simulink library "roller485lib"  (R2023a)
settings: Solver=VariableStepAuto  StartTime=0.0  StopTime=10.0  RelTol=1e-3
libraries: arduinolib x173, simulink x66
(part 5 of 6)

== system roller485lib/I2C Write/relative angle command [deg]/Enabled Subsystem (PID setting) ==
  P : Inport
  I : Inport  Port=2
  D : Inport  Port=3
  Enable : EnablePort
  " x 10^5 " : Gain  Gain=1e5
  Data Type Conversion1 : DataTypeConversion  OutDataTypeStr=uint32  SaturateOnIntegerOverflow=off  RndMeth=Floor
  Data Type Conversion2 : DataTypeConversion  OutDataTypeStr=uint32  SaturateOnIntegerOverflow=off  RndMeth=Floor
  Data Type Conversion3 : DataTypeConversion  OutDataTypeStr=uint32  SaturateOnIntegerOverflow=off  RndMeth=Floor
  I2C Write (0xA0) : arduinolib/I2C Write  I2CModule=0  Mode=Master  SlaveAddress=I2CAddress  SlaveByteOrder=LittleEndian  Direction=Transmitter  RegisterAddressMode=on  RegisterAddress=0xA0  SlaveDataType=uint8  DataLength=1  NoAck=off  RepeatedStart=off  OutputStatus=off  blockPlatform=ARDUINO
  I2C Write (0xA4) : arduinolib/I2C Write  I2CModule=0  Mode=Master  SlaveAddress=I2CAddress  SlaveByteOrder=LittleEndian  Direction=Transmitter  RegisterAddressMode=on  RegisterAddress=0xA4  SlaveDataType=uint8  DataLength=1  NoAck=off  RepeatedStart=off  OutputStatus=off  blockPlatform=ARDUINO
  I2C Write (0xA8) : arduinolib/I2C Write  I2CModule=0  Mode=Master  SlaveAddress=I2CAddress  SlaveByteOrder=LittleEndian  Direction=Transmitter  RegisterAddressMode=on  RegisterAddress=0xA8  SlaveDataType=uint8  DataLength=1  NoAck=off  RepeatedStart=off  OutputStatus=off  blockPlatform=ARDUINO
  x 10^5 : Gain  Gain=1e5
  x 10^7 : Gain  Gain=1e7
  wires:
  P/1 -> x 10^5/1
  I/1 -> x 10^7/1
  D/1 -> " x 10^5 "/1
  Data Type Conversion2/1 -> I2C Write (0xA4)/1
  Data Type Conversion3/1 -> I2C Write (0xA8)/1
  Data Type Conversion1/1 -> I2C Write (0xA0)/1
  x 10^5/1 -> Data Type Conversion1/1
  x 10^7/1 -> Data Type Conversion2/1
  " x 10^5 "/1 -> Data Type Conversion3/1

== system roller485lib/I2C Write/relative angle command [deg]/Enabled Subsystem (initialization angle) ==
  Enable : EnablePort
  Data Type Conversion : DataTypeConversion  OutDataTypeStr=double  SaturateOnIntegerOverflow=off  RndMeth=Floor
  I2C Read (0x90) : arduinolib/I2C Read  I2CModule=0  Mode=Master  SlaveAddress=I2CAddress  SlaveByteOrder=LittleEndian  Direction=Receiver  RegisterAddressMode=on  RegisterAddress=0x90  SlaveDataType=int32  DataLength=1  NoAck=off  RepeatedStart=off  OutputStatus=off  blockPlatform=ARDUINO  SampleTime=sample_time
  x (1/100) : Gain  Gain=1/100
  initial angle : Outport
  wires:
  I2C Read (0x90)/1 -> Data Type Conversion/1
  Data Type Conversion/1 -> x (1/100)/1
  x (1/100)/1 -> initial angle/1

== system roller485lib/I2C Write/relative angle command [deg]/Enabled Subsystem (mode setting) ==
  mode : Inport
  Enable : EnablePort
  Data Type Conversion : DataTypeConversion  OutDataTypeStr=uint8  SaturateOnIntegerOverflow=off  RndMeth=Floor
  I2C Write (0x01) : arduinolib/I2C Write  I2CModule=0  Mode=Master  SlaveAddress=I2CAddress  SlaveByteOrder=BigEndian  Direction=Transmitter  RegisterAddressMode=on  RegisterAddress=0x01  SlaveDataType=uint8  DataLength=1  NoAck=off  RepeatedStart=off  OutputStatus=off  blockPlatform=ARDUINO
  wires:
  Data Type Conversion/1 -> I2C Write (0x01)/1
  mode/1 -> Data Type Conversion/1

== system roller485lib/I2C Write/relative angle command [deg] and max current [mA]/Enabled Subsystem (PID setting) ==
  P : Inport
  I : Inport  Port=2
  D : Inport  Port=3
  Enable : EnablePort
  " x 10^5 " : Gain  Gain=1e5
  Data Type Conversion1 : DataTypeConversion  OutDataTypeStr=uint32  SaturateOnIntegerOverflow=off  RndMeth=Floor
  Data Type Conversion2 : DataTypeConversion  OutDataTypeStr=uint32  SaturateOnIntegerOverflow=off  RndMeth=Floor
  Data Type Conversion3 : DataTypeConversion  OutDataTypeStr=uint32  SaturateOnIntegerOverflow=off  RndMeth=Floor
  I2C Write (0xA0) : arduinolib/I2C Write  I2CModule=0  Mode=Master  SlaveAddress=I2CAddress  SlaveByteOrder=LittleEndian  Direction=Transmitter  RegisterAddressMode=on  RegisterAddress=0xA0  SlaveDataType=uint8  DataLength=1  NoAck=off  RepeatedStart=off  OutputStatus=off  blockPlatform=ARDUINO
  I2C Write (0xA4) : arduinolib/I2C Write  I2CModule=0  Mode=Master  SlaveAddress=I2CAddress  SlaveByteOrder=LittleEndian  Direction=Transmitter  RegisterAddressMode=on  RegisterAddress=0xA4  SlaveDataType=uint8  DataLength=1  NoAck=off  RepeatedStart=off  OutputStatus=off  blockPlatform=ARDUINO
  I2C Write (0xA8) : arduinolib/I2C Write  I2CModule=0  Mode=Master  SlaveAddress=I2CAddress  SlaveByteOrder=LittleEndian  Direction=Transmitter  RegisterAddressMode=on  RegisterAddress=0xA8  SlaveDataType=uint8  DataLength=1  NoAck=off  RepeatedStart=off  OutputStatus=off  blockPlatform=ARDUINO
  x 10^5 : Gain  Gain=1e5
  x 10^7 : Gain  Gain=1e7
  wires:
  P/1 -> x 10^5/1
  I/1 -> x 10^7/1
  D/1 -> " x 10^5 "/1
  Data Type Conversion2/1 -> I2C Write (0xA4)/1
  Data Type Conversion3/1 -> I2C Write (0xA8)/1
  Data Type Conversion1/1 -> I2C Write (0xA0)/1
  x 10^5/1 -> Data Type Conversion1/1
  x 10^7/1 -> Data Type Conversion2/1
  " x 10^5 "/1 -> Data Type Conversion3/1

== system roller485lib/I2C Write/relative angle command [deg] and max current [mA]/Enabled Subsystem (initialization angle) ==
  Enable : EnablePort
  Data Type Conversion : DataTypeConversion  OutDataTypeStr=double  SaturateOnIntegerOverflow=off  RndMeth=Floor
  I2C Read (0x90) : arduinolib/I2C Read  I2CModule=0  Mode=Master  SlaveAddress=I2CAddress  SlaveByteOrder=LittleEndian  Direction=Receiver  RegisterAddressMode=on  RegisterAddress=0x90  SlaveDataType=int32  DataLength=1  NoAck=off  RepeatedStart=off  OutputStatus=off  blockPlatform=ARDUINO  SampleTime=sample_time
  x (1/100) : Gain  Gain=1/100
  initial angle : Outport
  wires:
  I2C Read (0x90)/1 -> Data Type Conversion/1
  Data Type Conversion/1 -> x (1/100)/1
  x (1/100)/1 -> initial angle/1

== system roller485lib/I2C Write/relative angle command [deg] and max current [mA]/Enabled Subsystem (max current setting) ==
  max_current : Inport
  Enable : EnablePort
  Data Type Conversion : DataTypeConversion  OutDataTypeStr=uint32  SaturateOnIntegerOverflow=off  RndMeth=Floor
  I2C Write (0x50) : arduinolib/I2C Write  I2CModule=0  Mode=Master  SlaveAddress=I2CAddress  SlaveByteOrder=LittleEndian  Direction=Transmitter  RegisterAddressMode=on  RegisterAddress=0x50  SlaveDataType=uint8  DataLength=1  NoAck=off  RepeatedStart=off  OutputStatus=off  blockPlatform=ARDUINO
  x 100 : Gain  Gain=100
  wires:
  x 100/1 -> Data Type Conversion/1
  max_current/1 -> x 100/1
  Data Type Conversion/1 -> I2C Write (0x50)/1

== system roller485lib/I2C Write/relative angle command [deg] and max current [mA]/Enabled Subsystem (mode setting) ==
  mode : Inport
  Enable : EnablePort
  Data Type Conversion : DataTypeConversion  OutDataTypeStr=uint8  SaturateOnIntegerOverflow=off  RndMeth=Floor
  I2C Write (0x01) : arduinolib/I2C Write  I2CModule=0  Mode=Master  SlaveAddress=I2CAddress  SlaveByteOrder=BigEndian  Direction=Transmitter  RegisterAddressMode=on  RegisterAddress=0x01  SlaveDataType=uint8  DataLength=1  NoAck=off  RepeatedStart=off  OutputStatus=off  blockPlatform=ARDUINO
  wires:
  Data Type Conversion/1 -> I2C Write (0x01)/1
  mode/1 -> Data Type Conversion/1

== system roller485lib/I2C Write/relative angle command [rad]/Enabled Subsystem (PID setting) ==
  P : Inport
  I : Inport  Port=2
  D : Inport  Port=3
  Enable : EnablePort
  " x 10^5 " : Gain  Gain=1e5
  Data Type Conversion1 : DataTypeConversion  OutDataTypeStr=uint32  SaturateOnIntegerOverflow=off  RndMeth=Floor
  Data Type Conversion2 : DataTypeConversion  OutDataTypeStr=uint32  SaturateOnIntegerOverflow=off  RndMeth=Floor
  Data Type Conversion3 : DataTypeConversion  OutDataTypeStr=uint32  SaturateOnIntegerOverflow=off  RndMeth=Floor
  I2C Write (0xA0) : arduinolib/I2C Write  I2CModule=0  Mode=Master  SlaveAddress=I2CAddress  SlaveByteOrder=LittleEndian  Direction=Transmitter  RegisterAddressMode=on  RegisterAddress=0xA0  SlaveDataType=uint8  DataLength=1  NoAck=off  RepeatedStart=off  OutputStatus=off  blockPlatform=ARDUINO
  I2C Write (0xA4) : arduinolib/I2C Write  I2CModule=0  Mode=Master  SlaveAddress=I2CAddress  SlaveByteOrder=LittleEndian  Direction=Transmitter  RegisterAddressMode=on  RegisterAddress=0xA4  SlaveDataType=uint8  DataLength=1  NoAck=off  RepeatedStart=off  OutputStatus=off  blockPlatform=ARDUINO
  I2C Write (0xA8) : arduinolib/I2C Write  I2CModule=0  Mode=Master  SlaveAddress=I2CAddress  SlaveByteOrder=LittleEndian  Direction=Transmitter  RegisterAddressMode=on  RegisterAddress=0xA8  SlaveDataType=uint8  DataLength=1  NoAck=off  RepeatedStart=off  OutputStatus=off  blockPlatform=ARDUINO
  x 10^5 : Gain  Gain=1e5
  x 10^7 : Gain  Gain=1e7
  wires:
  P/1 -> x 10^5/1
  I/1 -> x 10^7/1
  D/1 -> " x 10^5 "/1
  Data Type Conversion2/1 -> I2C Write (0xA4)/1
  Data Type Conversion3/1 -> I2C Write (0xA8)/1
  Data Type Conversion1/1 -> I2C Write (0xA0)/1
  x 10^5/1 -> Data Type Conversion1/1
  x 10^7/1 -> Data Type Conversion2/1
  " x 10^5 "/1 -> Data Type Conversion3/1

== system roller485lib/I2C Write/relative angle command [rad]/Enabled Subsystem (initialization angle) ==
  Enable : EnablePort
  Data Type Conversion : DataTypeConversion  OutDataTypeStr=double  SaturateOnIntegerOverflow=off  RndMeth=Floor
  I2C Read (0x90) : arduinolib/I2C Read  I2CModule=0  Mode=Master  SlaveAddress=I2CAddress  SlaveByteOrder=LittleEndian  Direction=Receiver  RegisterAddressMode=on  RegisterAddress=0x90  SlaveDataType=int32  DataLength=1  NoAck=off  RepeatedStart=off  OutputStatus=off  blockPlatform=ARDUINO  SampleTime=sample_time
  x (1/100) : Gain  Gain=1/100
  initial angle : Outport
  wires:
  I2C Read (0x90)/1 -> Data Type Conversion/1
  Data Type Conversion/1 -> x (1/100)/1
  x (1/100)/1 -> initial angle/1

== system roller485lib/I2C Write/relative angle command [rad]/Enabled Subsystem (mode setting) ==
  mode : Inport
  Enable : EnablePort
  Data Type Conversion : DataTypeConversion  OutDataTypeStr=uint8  SaturateOnIntegerOverflow=off  RndMeth=Floor
  I2C Write (0x01) : arduinolib/I2C Write  I2CModule=0  Mode=Master  SlaveAddress=I2CAddress  SlaveByteOrder=BigEndian  Direction=Transmitter  RegisterAddressMode=on  RegisterAddress=0x01  SlaveDataType=uint8  DataLength=1  NoAck=off  RepeatedStart=off  OutputStatus=off  blockPlatform=ARDUINO
  wires:
  Data Type Conversion/1 -> I2C Write (0x01)/1
  mode/1 -> Data Type Conversion/1

== system roller485lib/I2C Write/relative angle command [rad] and max current [mA]/Enabled Subsystem (PID setting) ==
  P : Inport
  I : Inport  Port=2
  D : Inport  Port=3
  Enable : EnablePort
  " x 10^5 " : Gain  Gain=1e5
  Data Type Conversion1 : DataTypeConversion  OutDataTypeStr=uint32  SaturateOnIntegerOverflow=off  RndMeth=Floor
  Data Type Conversion2 : DataTypeConversion  OutDataTypeStr=uint32  SaturateOnIntegerOverflow=off  RndMeth=Floor
  Data Type Conversion3 : DataTypeConversion  OutDataTypeStr=uint32  SaturateOnIntegerOverflow=off  RndMeth=Floor
  I2C Write (0xA0) : arduinolib/I2C Write  I2CModule=0  Mode=Master  SlaveAddress=I2CAddress  SlaveByteOrder=LittleEndian  Direction=Transmitter  RegisterAddressMode=on  RegisterAddress=0xA0  SlaveDataType=uint8  DataLength=1  NoAck=off  RepeatedStart=off  OutputStatus=off  blockPlatform=ARDUINO
  I2C Write (0xA4) : arduinolib/I2C Write  I2CModule=0  Mode=Master  SlaveAddress=I2CAddress  SlaveByteOrder=LittleEndian  Direction=Transmitter  RegisterAddressMode=on  RegisterAddress=0xA4  SlaveDataType=uint8  DataLength=1  NoAck=off  RepeatedStart=off  OutputStatus=off  blockPlatform=ARDUINO
  I2C Write (0xA8) : arduinolib/I2C Write  I2CModule=0  Mode=Master  SlaveAddress=I2CAddress  SlaveByteOrder=LittleEndian  Direction=Transmitter  RegisterAddressMode=on  RegisterAddress=0xA8  SlaveDataType=uint8  DataLength=1  NoAck=off  RepeatedStart=off  OutputStatus=off  blockPlatform=ARDUINO
  x 10^5 : Gain  Gain=1e5
  x 10^7 : Gain  Gain=1e7
  wires:
  P/1 -> x 10^5/1
  I/1 -> x 10^7/1
  D/1 -> " x 10^5 "/1
  Data Type Conversion2/1 -> I2C Write (0xA4)/1
  Data Type Conversion3/1 -> I2C Write (0xA8)/1
  Data Type Conversion1/1 -> I2C Write (0xA0)/1
  x 10^5/1 -> Data Type Conversion1/1
  x 10^7/1 -> Data Type Conversion2/1
  " x 10^5 "/1 -> Data Type Conversion3/1

== system roller485lib/I2C Write/relative angle command [rad] and max current [mA]/Enabled Subsystem (initialization angle) ==
  Enable : EnablePort
  Data Type Conversion : DataTypeConversion  OutDataTypeStr=double  SaturateOnIntegerOverflow=off  RndMeth=Floor
  I2C Read (0x90) : arduinolib/I2C Read  I2CModule=0  Mode=Master  SlaveAddress=I2CAddress  SlaveByteOrder=LittleEndian  Direction=Receiver  RegisterAddressMode=on  RegisterAddress=0x90  SlaveDataType=int32  DataLength=1  NoAck=off  RepeatedStart=off  OutputStatus=off  blockPlatform=ARDUINO  SampleTime=sample_time
  x (1/100) : Gain  Gain=1/100
  initial angle : Outport
  wires:
  x (1/100)/1 -> initial angle/1
  Data Type Conversion/1 -> x (1/100)/1
  I2C Read (0x90)/1 -> Data Type Conversion/1

== system roller485lib/I2C Write/relative angle command [rad] and max current [mA]/Enabled Subsystem (max current setting) ==
  max_current : Inport
  Enable : EnablePort
  Data Type Conversion : DataTypeConversion  OutDataTypeStr=uint32  SaturateOnIntegerOverflow=off  RndMeth=Floor
  I2C Write (0x50) : arduinolib/I2C Write  I2CModule=0  Mode=Master  SlaveAddress=I2CAddress  SlaveByteOrder=LittleEndian  Direction=Transmitter  RegisterAddressMode=on  RegisterAddress=0x50  SlaveDataType=uint8  DataLength=1  NoAck=off  RepeatedStart=off  OutputStatus=off  blockPlatform=ARDUINO
  x 100 : Gain  Gain=100
  wires:
  x 100/1 -> Data Type Conversion/1
  max_current/1 -> x 100/1
  Data Type Conversion/1 -> I2C Write (0x50)/1

== system roller485lib/I2C Write/relative angle command [rad] and max current [mA]/Enabled Subsystem (mode setting) ==
  mode : Inport
  Enable : EnablePort
  Data Type Conversion : DataTypeConversion  OutDataTypeStr=uint8  SaturateOnIntegerOverflow=off  RndMeth=Floor
  I2C Write (0x01) : arduinolib/I2C Write  I2CModule=0  Mode=Master  SlaveAddress=I2CAddress  SlaveByteOrder=BigEndian  Direction=Transmitter  RegisterAddressMode=on  RegisterAddress=0x01  SlaveDataType=uint8  DataLength=1  NoAck=off  RepeatedStart=off  OutputStatus=off  blockPlatform=ARDUINO
  wires:
  Data Type Conversion/1 -> I2C Write (0x01)/1
  mode/1 -> Data Type Conversion/1

== system roller485lib/I2C Write (using MATLAB Function)/absolute angle command [deg] (using MATLAB Function)/Enabled Subsystem (PID setting) ==
  P : Inport
  I : Inport  Port=2
  D : Inport  Port=3
  Enable : EnablePort
  " x 10^5 " : Gain  Gain=1e5
  I2C Write (0xA0) : arduinolib/I2C Write  I2CModule=0  Mode=Master  SlaveAddress=I2CAddress  SlaveByteOrder=BigEndian  Direction=Transmitter  RegisterAddressMode=on  RegisterAddress=0xA0  SlaveDataType=uint8  DataLength=1  NoAck=off  RepeatedStart=off  OutputStatus=off  blockPlatform=ARDUINO
  I2C Write (0xA4) : arduinolib/I2C Write  I2CModule=0  Mode=Master  SlaveAddress=I2CAddress  SlaveByteOrder=BigEndian  Direction=Transmitter  RegisterAddressMode=on  RegisterAddress=0xA4  SlaveDataType=uint8  DataLength=1  NoAck=off  RepeatedStart=off  OutputStatus=off  blockPlatform=ARDUINO
  I2C Write (0xA8) : arduinolib/I2C Write  I2CModule=0  Mode=Master  SlaveAddress=I2CAddress  SlaveByteOrder=BigEndian  Direction=Transmitter  RegisterAddressMode=on  RegisterAddress=0xA8  SlaveDataType=uint8  DataLength=1  NoAck=off  RepeatedStart=off  OutputStatus=off  blockPlatform=ARDUINO
  MATLAB Function (D) : MATLAB Function  TreatAsAtomicUnit=on
  MATLAB Function (I) : MATLAB Function  TreatAsAtomicUnit=on
  MATLAB Function (P) : MATLAB Function  TreatAsAtomicUnit=on
  x 10^5 : Gain  Gain=1e5
  x 10^7 : Gain  Gain=1e7
  wires:
  x 10^7/1 -> MATLAB Function (I)/1(double_data)
  " x 10^5 "/1 -> MATLAB Function (D)/1(double_data)
  x 10^5/1 -> MATLAB Function (P)/1(double_data)
  P/1 -> x 10^5/1
  I/1 -> x 10^7/1
  D/1 -> " x 10^5 "/1
  MATLAB Function (P)/1(bytes) -> I2C Write (0xA0)/1
  MATLAB Function (D)/1(bytes) -> I2C Write (0xA8)/1
  MATLAB Function (I)/1(bytes) -> I2C Write (0xA4)/1

== system roller485lib/I2C Write (using MATLAB Function)/absolute angle command [deg] (using MATLAB Function)/Enabled Subsystem (mode setting) ==
  mode : Inport
  Enable : EnablePort
  Data Type Conversion : DataTypeConversion  OutDataTypeStr=uint8  SaturateOnIntegerOverflow=off  RndMeth=Floor
  I2C Write (0x01) : arduinolib/I2C Write  I2CModule=0  Mode=Master  SlaveAddress=I2CAddress  SlaveByteOrder=BigEndian  Direction=Transmitter  RegisterAddressMode=on  RegisterAddress=0x01  SlaveDataType=uint8  DataLength=1  NoAck=off  RepeatedStart=off  OutputStatus=off  blockPlatform=ARDUINO
  wires:
  Data Type Conversion/1 -> I2C Write (0x01)/1
  mode/1 -> Data Type Conversion/1

== system roller485lib/I2C Write (using MATLAB Function)/absolute angle command [rad] (using MATLAB Function)/Enabled Subsystem (PID setting) ==
  P : Inport
  I : Inport  Port=2
  D : Inport  Port=3
  Enable : EnablePort
  " x 10^5 " : Gain  Gain=1e5
  I2C Write (0xA0) : arduinolib/I2C Write  I2CModule=0  Mode=Master  SlaveAddress=I2CAddress  SlaveByteOrder=BigEndian  Direction=Transmitter  RegisterAddressMode=on  RegisterAddress=0xA0  SlaveDataType=uint8  DataLength=1  NoAck=off  RepeatedStart=off  OutputStatus=off  blockPlatform=ARDUINO
  I2C Write (0xA4) : arduinolib/I2C Write  I2CModule=0  Mode=Master  SlaveAddress=I2CAddress  SlaveByteOrder=BigEndian  Direction=Transmitter  RegisterAddressMode=on  RegisterAddress=0xA4  SlaveDataType=uint8  DataLength=1  NoAck=off  RepeatedStart=off  OutputStatus=off  blockPlatform=ARDUINO
  I2C Write (0xA8) : arduinolib/I2C Write  I2CModule=0  Mode=Master  SlaveAddress=I2CAddress  SlaveByteOrder=BigEndian  Direction=Transmitter  RegisterAddressMode=on  RegisterAddress=0xA8  SlaveDataType=uint8  DataLength=1  NoAck=off  RepeatedStart=off  OutputStatus=off  blockPlatform=ARDUINO
  MATLAB Function (D) : MATLAB Function  TreatAsAtomicUnit=on
  MATLAB Function (I) : MATLAB Function  TreatAsAtomicUnit=on
  MATLAB Function (P) : MATLAB Function  TreatAsAtomicUnit=on
  x 10^5 : Gain  Gain=1e5
  x 10^7 : Gain  Gain=1e7
  wires:
  x 10^7/1 -> MATLAB Function (I)/1(double_data)
  " x 10^5 "/1 -> MATLAB Function (D)/1(double_data)
  x 10^5/1 -> MATLAB Function (P)/1(double_data)
  P/1 -> x 10^5/1
  I/1 -> x 10^7/1
  D/1 -> " x 10^5 "/1
  MATLAB Function (P)/1(bytes) -> I2C Write (0xA0)/1
  MATLAB Function (D)/1(bytes) -> I2C Write (0xA8)/1
  MATLAB Function (I)/1(bytes) -> I2C Write (0xA4)/1

== system roller485lib/I2C Write (using MATLAB Function)/absolute angle command [rad] (using MATLAB Function)/Enabled Subsystem (mode setting) ==
  mode : Inport
  Enable : EnablePort
  Data Type Conversion : DataTypeConversion  OutDataTypeStr=uint8  SaturateOnIntegerOverflow=off  RndMeth=Floor
  I2C Write (0x01) : arduinolib/I2C Write  I2CModule=0  Mode=Master  SlaveAddress=I2CAddress  SlaveByteOrder=BigEndian  Direction=Transmitter  RegisterAddressMode=on  RegisterAddress=0x01  SlaveDataType=uint8  DataLength=1  NoAck=off  RepeatedStart=off  OutputStatus=off  blockPlatform=ARDUINO
  wires:
  mode/1 -> Data Type Conversion/1
  Data Type Conversion/1 -> I2C Write (0x01)/1

== system roller485lib/I2C Write (using MATLAB Function)/angular velocity command [rad//s] (using MATLAB Function)/Enabled Subsystem (PID setting) ==
  P : Inport
  I : Inport  Port=2
  D : Inport  Port=3
  Enable : EnablePort
  " x 10^5 " : Gain  Gain=1e5
  I2C Write (0x70) : arduinolib/I2C Write  I2CModule=0  Mode=Master  SlaveAddress=I2CAddress  SlaveByteOrder=BigEndian  Direction=Transmitter  RegisterAddressMode=on  RegisterAddress=0x70  SlaveDataType=uint8  DataLength=1  NoAck=off  RepeatedStart=off  OutputStatus=off  blockPlatform=ARDUINO
  I2C Write (0x74) : arduinolib/I2C Write  I2CModule=0  Mode=Master  SlaveAddress=I2CAddress  SlaveByteOrder=BigEndian  Direction=Transmitter  RegisterAddressMode=on  RegisterAddress=0x74  SlaveDataType=uint8  DataLength=1  NoAck=off  RepeatedStart=off  OutputStatus=off  blockPlatform=ARDUINO
  I2C Write (0x78) : arduinolib/I2C Write  I2CModule=0  Mode=Master  SlaveAddress=I2CAddress  SlaveByteOrder=BigEndian  Direction=Transmitter  RegisterAddressMode=on  RegisterAddress=0x78  SlaveDataType=uint8  DataLength=1  NoAck=off  RepeatedStart=off  OutputStatus=off  blockPlatform=ARDUINO
  MATLAB Function (D) : MATLAB Function  TreatAsAtomicUnit=on
  MATLAB Function (I) : MATLAB Function  TreatAsAtomicUnit=on
  MATLAB Function (P) : MATLAB Function  TreatAsAtomicUnit=on
  x 10^5 : Gain  Gain=1e5
  x 10^7 : Gain  Gain=1e7
  wires:
  P/1 -> x 10^5/1
  I/1 -> x 10^7/1
  D/1 -> " x 10^5 "/1
  x 10^5/1 -> MATLAB Function (P)/1(double_data)
  x 10^7/1 -> MATLAB Function (I)/1(double_data)
  " x 10^5 "/1 -> MATLAB Function (D)/1(double_data)
  MATLAB Function (P)/1(bytes) -> I2C Write (0x70)/1
  MATLAB Function (I)/1(bytes) -> I2C Write (0x74)/1
  MATLAB Function (D)/1(bytes) -> I2C Write (0x78)/1

== system roller485lib/I2C Write (using MATLAB Function)/angular velocity command [rad//s] (using MATLAB Function)/Enabled Subsystem (mode setting) ==
  mode : Inport
  Enable : EnablePort
  Data Type Conversion : DataTypeConversion  OutDataTypeStr=uint8  SaturateOnIntegerOverflow=off  RndMeth=Floor
  I2C Write (0x01) : arduinolib/I2C Write  I2CModule=0  Mode=Master  SlaveAddress=I2CAddress  SlaveByteOrder=BigEndian  Direction=Transmitter  RegisterAddressMode=on  RegisterAddress=0x01  SlaveDataType=uint8  DataLength=1  NoAck=off  RepeatedStart=off  OutputStatus=off  blockPlatform=ARDUINO
  wires:
  mode/1 -> Data Type Conversion/1
  Data Type Conversion/1 -> I2C Write (0x01)/1

== system roller485lib/I2C Write (using MATLAB Function)/angular velocity command [rpm] (using MATLAB Function)/Enabled Subsystem (PID setting) ==
  P : Inport
  I : Inport  Port=2
  D : Inport  Port=3
  Enable : EnablePort
  " x 10^5 " : Gain  Gain=1e5
  I2C Write (0x70) : arduinolib/I2C Write  I2CModule=0  Mode=Master  SlaveAddress=I2CAddress  SlaveByteOrder=BigEndian  Direction=Transmitter  RegisterAddressMode=on  RegisterAddress=0x70  SlaveDataType=uint8  DataLength=1  NoAck=off  RepeatedStart=off  OutputStatus=off  blockPlatform=ARDUINO
  I2C Write (0x74) : arduinolib/I2C Write  I2CModule=0  Mode=Master  SlaveAddress=I2CAddress  SlaveByteOrder=BigEndian  Direction=Transmitter  RegisterAddressMode=on  RegisterAddress=0x74  SlaveDataType=uint8  DataLength=1  NoAck=off  RepeatedStart=off  OutputStatus=off  blockPlatform=ARDUINO
  I2C Write (0x78) : arduinolib/I2C Write  I2CModule=0  Mode=Master  SlaveAddress=I2CAddress  SlaveByteOrder=BigEndian  Direction=Transmitter  RegisterAddressMode=on  RegisterAddress=0x78  SlaveDataType=uint8  DataLength=1  NoAck=off  RepeatedStart=off  OutputStatus=off  blockPlatform=ARDUINO
  MATLAB Function (D) : MATLAB Function  TreatAsAtomicUnit=on
  MATLAB Function (I) : MATLAB Function  TreatAsAtomicUnit=on
  MATLAB Function (P) : MATLAB Function  TreatAsAtomicUnit=on
  x 10^5 : Gain  Gain=1e5
  x 10^7 : Gain  Gain=1e7
  wires:
  P/1 -> x 10^5/1
  I/1 -> x 10^7/1
  D/1 -> " x 10^5 "/1
  x 10^5/1 -> MATLAB Function (P)/1(double_data)
  x 10^7/1 -> MATLAB Function (I)/1(double_data)
  " x 10^5 "/1 -> MATLAB Function (D)/1(double_data)
  MATLAB Function (P)/1(bytes) -> I2C Write (0x70)/1
  MATLAB Function (I)/1(bytes) -> I2C Write (0x74)/1
  MATLAB Function (D)/1(bytes) -> I2C Write (0x78)/1

== system roller485lib/I2C Write (using MATLAB Function)/angular velocity command [rpm] (using MATLAB Function)/Enabled Subsystem (mode setting) ==
  mode : Inport
  Enable : EnablePort
  Data Type Conversion : DataTypeConversion  OutDataTypeStr=uint8  SaturateOnIntegerOverflow=off  RndMeth=Floor
  I2C Write (0x01) : arduinolib/I2C Write  I2CModule=0  Mode=Master  SlaveAddress=I2CAddress  SlaveByteOrder=BigEndian  Direction=Transmitter  RegisterAddressMode=on  RegisterAddress=0x01  SlaveDataType=uint8  DataLength=1  NoAck=off  RepeatedStart=off  OutputStatus=off  blockPlatform=ARDUINO
  wires:
  Data Type Conversion/1 -> I2C Write (0x01)/1
  mode/1 -> Data Type Conversion/1

== system roller485lib/I2C Write (using MATLAB Function)/current command [A] (using MATLAB Function)/Enabled Subsystem (mode setting) ==
  mode : Inport
  Enable : EnablePort
  Data Type Conversion : DataTypeConversion  OutDataTypeStr=uint8  SaturateOnIntegerOverflow=off  RndMeth=Floor
  I2C Write (0x01) : arduinolib/I2C Write  I2CModule=0  Mode=Master  SlaveAddress=I2CAddress  SlaveByteOrder=BigEndian  Direction=Transmitter  RegisterAddressMode=on  RegisterAddress=0x01  SlaveDataType=uint8  DataLength=1  NoAck=off  RepeatedStart=off  OutputStatus=off  blockPlatform=ARDUINO
  wires:
  mode/1 -> Data Type Conversion/1
  Data Type Conversion/1 -> I2C Write (0x01)/1

== system roller485lib/I2C Write (using MATLAB Function)/current command [mA] (using MATLAB Function)/Enabled Subsystem (mode setting) ==
  mode : Inport
  Enable : EnablePort
  Data Type Conversion : DataTypeConversion  OutDataTypeStr=uint8  SaturateOnIntegerOverflow=off  RndMeth=Floor
  I2C Write (0x01) : arduinolib/I2C Write  I2CModule=0  Mode=Master  SlaveAddress=I2CAddress  SlaveByteOrder=BigEndian  Direction=Transmitter  RegisterAddressMode=on  RegisterAddress=0x01  SlaveDataType=uint8  DataLength=1  NoAck=off  RepeatedStart=off  OutputStatus=off  blockPlatform=ARDUINO
  wires:
  Data Type Conversion/1 -> I2C Write (0x01)/1
  mode/1 -> Data Type Conversion/1

== system roller485lib/I2C Write (using MATLAB Function)/relative angle command [deg] (using MATLAB Function)/Enabled Subsystem (PID setting) ==
  P : Inport
  I : Inport  Port=2
  D : Inport  Port=3
  Enable : EnablePort
  " x 10^5 " : Gain  Gain=1e5
  I2C Write (0xA0) : arduinolib/I2C Write  I2CModule=0  Mode=Master  SlaveAddress=I2CAddress  SlaveByteOrder=BigEndian  Direction=Transmitter  RegisterAddressMode=on  RegisterAddress=0xA0  SlaveDataType=uint8  DataLength=1  NoAck=off  RepeatedStart=off  OutputStatus=off  blockPlatform=ARDUINO
  I2C Write (0xA4) : arduinolib/I2C Write  I2CModule=0  Mode=Master  SlaveAddress=I2CAddress  SlaveByteOrder=BigEndian  Direction=Transmitter  RegisterAddressMode=on  RegisterAddress=0xA4  SlaveDataType=uint8  DataLength=1  NoAck=off  RepeatedStart=off  OutputStatus=off  blockPlatform=ARDUINO
  I2C Write (0xA8) : arduinolib/I2C Write  I2CModule=0  Mode=Master  SlaveAddress=I2CAddress  SlaveByteOrder=BigEndian  Direction=Transmitter  RegisterAddressMode=on  RegisterAddress=0xA8  SlaveDataType=uint8  DataLength=1  NoAck=off  RepeatedStart=off  OutputStatus=off  blockPlatform=ARDUINO
  MATLAB Function (D) : MATLAB Function  TreatAsAtomicUnit=on
  MATLAB Function (I) : MATLAB Function  TreatAsAtomicUnit=on
  MATLAB Function (P) : MATLAB Function  TreatAsAtomicUnit=on
  x 10^5 : Gain  Gain=1e5
  x 10^7 : Gain  Gain=1e7
  wires:
  x 10^7/1 -> MATLAB Function (I)/1(double_data)
  " x 10^5 "/1 -> MATLAB Function (D)/1(double_data)
  x 10^5/1 -> MATLAB Function (P)/1(double_data)
  P/1 -> x 10^5/1
  I/1 -> x 10^7/1
  D/1 -> " x 10^5 "/1
  MATLAB Function (P)/1(bytes) -> I2C Write (0xA0)/1
  MATLAB Function (D)/1(bytes) -> I2C Write (0xA8)/1
  MATLAB Function (I)/1(bytes) -> I2C Write (0xA4)/1

== system roller485lib/I2C Write (using MATLAB Function)/relative angle command [deg] (using MATLAB Function)/Enabled Subsystem (initialization angle) ==
  Enable : EnablePort
  I2C Read (0x90) : arduinolib/I2C Read  I2CModule=0  Mode=Master  SlaveAddress=0x64  SlaveByteOrder=BigEndian  Direction=Receiver  RegisterAddressMode=on  RegisterAddress=0x90  SlaveDataType=uint8  DataLength=4  NoAck=off  RepeatedStart=off  OutputStatus=off  blockPlatform=ARDUINO  SampleTime=sample_time
  MATLAB Function : MATLAB Function  TreatAsAtomicUnit=on
  x (1/100) : Gain  Gain=1/100
  initial angle : Outport
  wires:
  x (1/100)/1 -> initial angle/1
  I2C Read (0x90)/1 -> MATLAB Function/1(bytes)
  MATLAB Function/1(double_data) -> x (1/100)/1

== system roller485lib/I2C Write (using MATLAB Function)/relative angle command [deg] (using MATLAB Function)/Enabled Subsystem (mode setting) ==
  mode : Inport
  Enable : EnablePort
  Data Type Conversion : DataTypeConversion  OutDataTypeStr=uint8  SaturateOnIntegerOverflow=off  RndMeth=Floor
  I2C Write (0x01) : arduinolib/I2C Write  I2CModule=0  Mode=Master  SlaveAddress=I2CAddress  SlaveByteOrder=BigEndian  Direction=Transmitter  RegisterAddressMode=on  RegisterAddress=0x01  SlaveDataType=uint8  DataLength=1  NoAck=off  RepeatedStart=off  OutputStatus=off  blockPlatform=ARDUINO
  wires:
  Data Type Conversion/1 -> I2C Write (0x01)/1
  mode/1 -> Data Type Conversion/1

== system roller485lib/I2C Write (using MATLAB Function)/relative angle command [rad] (using MATLAB Function)/Enabled Subsystem (PID setting) ==
  P : Inport
  I : Inport  Port=2
  D : Inport  Port=3
  Enable : EnablePort
  " x 10^5 " : Gain  Gain=1e5
  I2C Write (0xA0) : arduinolib/I2C Write  I2CModule=0  Mode=Master  SlaveAddress=I2CAddress  SlaveByteOrder=BigEndian  Direction=Transmitter  RegisterAddressMode=on  RegisterAddress=0xA0  SlaveDataType=uint8  DataLength=1  NoAck=off  RepeatedStart=off  OutputStatus=off  blockPlatform=ARDUINO
  I2C Write (0xA4) : arduinolib/I2C Write  I2CModule=0  Mode=Master  SlaveAddress=I2CAddress  SlaveByteOrder=BigEndian  Direction=Transmitter  RegisterAddressMode=on  RegisterAddress=0xA4  SlaveDataType=uint8  DataLength=1  NoAck=off  RepeatedStart=off  OutputStatus=off  blockPlatform=ARDUINO
  I2C Write (0xA8) : arduinolib/I2C Write  I2CModule=0  Mode=Master  SlaveAddress=I2CAddress  SlaveByteOrder=BigEndian  Direction=Transmitter  RegisterAddressMode=on  RegisterAddress=0xA8  SlaveDataType=uint8  DataLength=1  NoAck=off  RepeatedStart=off  OutputStatus=off  blockPlatform=ARDUINO
  MATLAB Function (D) : MATLAB Function  TreatAsAtomicUnit=on
  MATLAB Function (I) : MATLAB Function  TreatAsAtomicUnit=on
  MATLAB Function (P) : MATLAB Function  TreatAsAtomicUnit=on
  x 10^5 : Gain  Gain=1e5
  x 10^7 : Gain  Gain=1e7
  wires:
  x 10^7/1 -> MATLAB Function (I)/1(double_data)
  " x 10^5 "/1 -> MATLAB Function (D)/1(double_data)
  x 10^5/1 -> MATLAB Function (P)/1(double_data)
  P/1 -> x 10^5/1
  I/1 -> x 10^7/1
  D/1 -> " x 10^5 "/1
  MATLAB Function (P)/1(bytes) -> I2C Write (0xA0)/1
  MATLAB Function (D)/1(bytes) -> I2C Write (0xA8)/1
  MATLAB Function (I)/1(bytes) -> I2C Write (0xA4)/1

== system roller485lib/I2C Write (using MATLAB Function)/relative angle command [rad] (using MATLAB Function)/Enabled Subsystem (initialization angle) ==
  Enable : EnablePort
  I2C Read (0x90) : arduinolib/I2C Read  I2CModule=0  Mode=Master  SlaveAddress=0x64  SlaveByteOrder=BigEndian  Direction=Receiver  RegisterAddressMode=on  RegisterAddress=0x90  SlaveDataType=uint8  DataLength=4  NoAck=off  RepeatedStart=off  OutputStatus=off  blockPlatform=ARDUINO  SampleTime=sample_time
  MATLAB Function : MATLAB Function  TreatAsAtomicUnit=on
  x (1/100) : Gain  Gain=1/100
  initial angle : Outport
  wires:
  MATLAB Function/1(double_data) -> x (1/100)/1
  I2C Read (0x90)/1 -> MATLAB Function/1(bytes)
  x (1/100)/1 -> initial angle/1

== system roller485lib/I2C Write (using MATLAB Function)/relative angle command [rad] (using MATLAB Function)/Enabled Subsystem (mode setting) ==
  mode : Inport
  Enable : EnablePort
  Data Type Conversion : DataTypeConversion  OutDataTypeStr=uint8  SaturateOnIntegerOverflow=off  RndMeth=Floor
  I2C Write (0x01) : arduinolib/I2C Write  I2CModule=0  Mode=Master  SlaveAddress=I2CAddress  SlaveByteOrder=BigEndian  Direction=Transmitter  RegisterAddressMode=on  RegisterAddress=0x01  SlaveDataType=uint8  DataLength=1  NoAck=off  RepeatedStart=off  OutputStatus=off  blockPlatform=ARDUINO
  wires:
  mode/1 -> Data Type Conversion/1
  Data Type Conversion/1 -> I2C Write (0x01)/1

== matlab function roller485lib/I2C Write (using MATLAB Function)/absolute angle command [deg] (using MATLAB Function)/MATLAB Function ==
  data: double_data input; bytes output
function bytes = double_to_bytes_uint8(double_data)

bytes        = zeros(1, 4, 'uint8');             % 明示的に型とサイズを宣言
signed_int   = int32(double_data);
unsigned_int = typecast(signed_int, 'uint32');
bytes(1:4)   = typecast(unsigned_int, 'uint8');  % サイズを明示

== matlab function roller485lib/I2C Write (using MATLAB Function)/absolute angle command [rad] (using MATLAB Function)/MATLAB Function ==
  data: double_data input; bytes output
function bytes = double_to_bytes_uint8(double_data)

bytes        = zeros(1, 4, 'uint8');             % 明示的に型とサイズを宣言
signed_int   = int32(double_data);
unsigned_int = typecast(signed_int, 'uint32');
bytes(1:4)   = typecast(unsigned_int, 'uint8');  % サイズを明示

== matlab function roller485lib/I2C Write (using MATLAB Function)/angular velocity command [rad//s] (using MATLAB Function)/MATLAB Function ==
  data: double_data input; bytes output
function bytes = double_to_bytes_uint8(double_data)

bytes        = zeros(1, 4, 'uint8');             % 明示的に型とサイズを宣言
signed_int   = int32(double_data);
unsigned_int = typecast(signed_int, 'uint32');
bytes(1:4)   = typecast(unsigned_int, 'uint8');  % サイズを明示

== matlab function roller485lib/I2C Write (using MATLAB Function)/angular velocity command [rpm] (using MATLAB Function)/MATLAB Function ==
  data: double_data input; bytes output
function bytes = double_to_bytes_uint8(double_data)

bytes        = zeros(1, 4, 'uint8');             % 明示的に型とサイズを宣言
signed_int   = int32(double_data);
unsigned_int = typecast(signed_int, 'uint32');
bytes(1:4)   = typecast(unsigned_int, 'uint8');  % サイズを明示

== matlab function roller485lib/I2C Write (using MATLAB Function)/current command [A] (using MATLAB Function)/MATLAB Function ==
  data: double_data input; bytes output
function bytes = double_to_bytes_uint8(double_data)

bytes        = zeros(1, 4, 'uint8');             % 明示的に型とサイズを宣言
signed_int   = int32(double_data);
unsigned_int = typecast(signed_int, 'uint32');
bytes(1:4)   = typecast(unsigned_int, 'uint8');  % サイズを明示

== matlab function roller485lib/I2C Write (using MATLAB Function)/current command [mA] (using MATLAB Function)/MATLAB Function ==
  data: double_data input; bytes output
function bytes = double_to_bytes_uint8(double_data)

bytes        = zeros(1, 4, 'uint8');             % 明示的に型とサイズを宣言
signed_int   = int32(double_data);
unsigned_int = typecast(signed_int, 'uint32');
bytes(1:4)   = typecast(unsigned_int, 'uint8');  % サイズを明示

== matlab function roller485lib/I2C Write (using MATLAB Function)/relative angle command [deg] (using MATLAB Function)/Enabled Subsystem (initialization angle)/MATLAB Function ==
  data: bytes input; double_data output
function double_data = bytes_uint8_to_double(bytes)

double_data    = zeros(1, 1, 'double');    % 明示的に型とサイズを宣言
unsigned_int   = typecast(uint8(bytes), 'uint32');
signed_int     = typecast(unsigned_int, 'int32');
double_data(1) = double(signed_int);       % サイズを明示

== matlab function roller485lib/I2C Write (using MATLAB Function)/relative angle command [deg] (using MATLAB Function)/MATLAB Function ==
  data: double_data input; bytes output
function bytes = double_to_bytes_uint8(double_data)

bytes        = zeros(1, 4, 'uint8');             % 明示的に型とサイズを宣言
signed_int   = int32(double_data);
unsigned_int = typecast(signed_int, 'uint32');
bytes(1:4)   = typecast(unsigned_int, 'uint8');  % サイズを明示

== matlab function roller485lib/I2C Write (using MATLAB Function)/relative angle command [rad] (using MATLAB Function)/Enabled Subsystem (initialization angle)/MATLAB Function ==
  data: bytes input; double_data output
function double_data = bytes_uint8_to_double(bytes)

double_data    = zeros(1, 1, 'double');    % 明示的に型とサイズを宣言
unsigned_int   = typecast(uint8(bytes), 'uint32');
signed_int     = typecast(unsigned_int, 'int32');
double_data(1) = double(signed_int);       % サイズを明示

== matlab function roller485lib/I2C Write (using MATLAB Function)/relative angle command [rad] (using MATLAB Function)/MATLAB Function ==
  data: double_data input; bytes output
function bytes = double_to_bytes_uint8(double_data)

bytes        = zeros(1, 4, 'uint8');             % 明示的に型とサイズを宣言
signed_int   = int32(double_data);
unsigned_int = typecast(signed_int, 'uint32');
bytes(1:4)   = typecast(unsigned_int, 'uint8');  % サイズを明示

== matlab function roller485lib/I2C Read (using MATLAB Function)/absolute angle detection [rad] (using MATLAB Function)/MATLAB Function ==
  data: bytes input; double_data output
function double_data = bytes_uint8_to_double(bytes)

double_data    = zeros(1, 1, 'double');    % 明示的に型とサイズを宣言
unsigned_int   = typecast(uint8(bytes), 'uint32');
signed_int     = typecast(unsigned_int, 'int32');
double_data(1) = double(signed_int);       % サイズを明示

== matlab function roller485lib/I2C Read (using MATLAB Function)/relative angle detection [rad] (using MATLAB Function)/MATLAB Function ==
  data: bytes input; double_data output
function double_data = bytes_uint8_to_double(bytes)

double_data    = zeros(1, 1, 'double');    % 明示的に型とサイズを宣言
unsigned_int   = typecast(uint8(bytes), 'uint32');
signed_int     = typecast(unsigned_int, 'int32');
double_data(1) = double(signed_int);       % サイズを明示

== matlab function roller485lib/I2C Read (using MATLAB Function)/absolute angle detection [deg] (using MATLAB Function)/MATLAB Function ==
  data: bytes input; double_data output
function double_data = bytes_uint8_to_double(bytes)

double_data    = zeros(1, 1, 'double');    % 明示的に型とサイズを宣言
unsigned_int   = typecast(uint8(bytes), 'uint32');
signed_int     = typecast(unsigned_int, 'int32');
double_data(1) = double(signed_int);       % サイズを明示

== matlab function roller485lib/I2C Read (using MATLAB Function)/angular velocity detection using LPF [rpm] (using MATLAB Function)/MATLAB Function2 ==
  data: bytes input; double_data output
function double_data = bytes_uint8_to_double(bytes)

double_data    = zeros(1, 1, 'double');    % 明示的に型とサイズを宣言
unsigned_int   = typecast(uint8(bytes), 'uint32');
signed_int     = typecast(unsigned_int, 'int32');
double_data(1) = double(signed_int);       % サイズを明示

== matlab function roller485lib/I2C Read (using MATLAB Function)/current detection [mA] (using MATLAB Function)/MATLAB Function ==
  data: bytes input; double_data output
function double_data = bytes_uint8_to_double(bytes)

double_data    = zeros(1, 1, 'double');    % 明示的に型とサイズを宣言
unsigned_int   = typecast(uint8(bytes), 'uint32');
signed_int     = typecast(unsigned_int, 'int32');
double_data(1) = double(signed_int);       % サイズを明示

== matlab function roller485lib/I2C Read (using MATLAB Function)/angular velocity detection using LPF [rad//s] (using MATLAB Function)/MATLAB Function2 ==
  data: bytes input; double_data output
function double_data = bytes_uint8_to_double(bytes)

double_data    = zeros(1, 1, 'double');    % 明示的に型とサイズを宣言
unsigned_int   = typecast(uint8(bytes), 'uint32');
signed_int     = typecast(unsigned_int, 'int32');
double_data(1) = double(signed_int);       % サイズを明示

== matlab function roller485lib/I2C Read (using MATLAB Function)/relative angle detection [deg] (using MATLAB Function)/MATLAB Function ==
  data: bytes input; double_data output
function double_data = bytes_uint8_to_double(bytes)

double_data    = zeros(1, 1, 'double');    % 明示的に型とサイズを宣言
unsigned_int   = typecast(uint8(bytes), 'uint32');
signed_int     = typecast(unsigned_int, 'int32');
double_data(1) = double(signed_int);       % サイズを明示

== matlab function roller485lib/Basic I2C Write (using MATLAB Function)/basic relative angle command [rad] (using MATLAB Function)/Enabled Subsystem (initialization angle)/MATLAB Function ==
  data: bytes input; double_data output
function double_data = bytes_uint8_to_double(bytes)

double_data    = zeros(1, 1, 'double');    % 明示的に型とサイズを宣言
unsigned_int   = typecast(uint8(bytes), 'uint32');
signed_int     = typecast(unsigned_int, 'int32');
double_data(1) = double(signed_int);       % サイズを明示

== matlab function roller485lib/Basic I2C Write (using MATLAB Function)/basic relative angle command [rad] (using MATLAB Function)/MATLAB Function ==
  data: double_data input; bytes output
function bytes = double_to_bytes_uint8(double_data)

bytes        = zeros(1, 4, 'uint8');             % 明示的に型とサイズを宣言
signed_int   = int32(double_data);
unsigned_int = typecast(signed_int, 'uint32');
bytes(1:4)   = typecast(unsigned_int, 'uint8');  % サイズを明示

== matlab function roller485lib/Basic I2C Write (using MATLAB Function)/position PID (using MATLAB Function)/MATLAB Function (D) ==
  data: double_data input; bytes output
function bytes = double_to_bytes_uint8(double_data)

bytes        = zeros(1, 4, 'uint8');             % 明示的に型とサイズを宣言
signed_int   = int32(double_data);
unsigned_int = typecast(signed_int, 'uint32');
bytes(1:4)   = typecast(unsigned_int, 'uint8');  % サイズを明示

== matlab function roller485lib/Basic I2C Write (using MATLAB Function)/position PID (using MATLAB Function)/MATLAB Function (I) ==
  data: double_data input; bytes output
function bytes = double_to_bytes_uint8(double_data)

bytes        = zeros(1, 4, 'uint8');             % 明示的に型とサイズを宣言
signed_int   = int32(double_data);
unsigned_int = typecast(signed_int, 'uint32');
bytes(1:4)   = typecast(unsigned_int, 'uint8');  % サイズを明示

== matlab function roller485lib/Basic I2C Write (using MATLAB Function)/position PID (using MATLAB Function)/MATLAB Function (P) ==
  data: double_data input; bytes output
function bytes = double_to_bytes_uint8(double_data)

bytes        = zeros(1, 4, 'uint8');             % 明示的に型とサイズを宣言
signed_int   = int32(double_data);
unsigned_int = typecast(signed_int, 'uint32');
bytes(1:4)   = typecast(unsigned_int, 'uint8');  % サイズを明示

== matlab function roller485lib/Basic I2C Write (using MATLAB Function)/position PID (within set time) (using MATLAB Function)/Enabled Subsystem/MATLAB Function (D) ==
  data: double_data input; bytes output
function bytes = double_to_bytes_uint8(double_data)

bytes        = zeros(1, 4, 'uint8');             % 明示的に型とサイズを宣言
signed_int   = int32(double_data);
unsigned_int = typecast(signed_int, 'uint32');
bytes(1:4)   = typecast(unsigned_int, 'uint8');  % サイズを明示

== matlab function roller485lib/Basic I2C Write (using MATLAB Function)/position PID (within set time) (using MATLAB Function)/Enabled Subsystem/MATLAB Function (I) ==
  data: double_data input; bytes output
function bytes = double_to_bytes_uint8(double_data)

bytes        = zeros(1, 4, 'uint8');             % 明示的に型とサイズを宣言
signed_int   = int32(double_data);
unsigned_int = typecast(signed_int, 'uint32');
bytes(1:4)   = typecast(unsigned_int, 'uint8');  % サイズを明示

== matlab function roller485lib/Basic I2C Write (using MATLAB Function)/position PID (within set time) (using MATLAB Function)/Enabled Subsystem/MATLAB Function (P) ==
  data: double_data input; bytes output
function bytes = double_to_bytes_uint8(double_data)

bytes        = zeros(1, 4, 'uint8');             % 明示的に型とサイズを宣言
signed_int   = int32(double_data);
unsigned_int = typecast(signed_int, 'uint32');
bytes(1:4)   = typecast(unsigned_int, 'uint8');  % サイズを明示

== matlab function roller485lib/Basic I2C Write (using MATLAB Function)/speed PID (using MATLAB Function)/MATLAB Function (D) ==
  data: double_data input; bytes output
function bytes = double_to_bytes_uint8(double_data)

bytes        = zeros(1, 4, 'uint8');             % 明示的に型とサイズを宣言
signed_int   = int32(double_data);
unsigned_int = typecast(signed_int, 'uint32');
bytes(1:4)   = typecast(unsigned_int, 'uint8');  % サイズを明示

== matlab function roller485lib/I2C Read (using MATLAB Function)/current detection [A] (using MATLAB Function)/MATLAB Function ==
  data: bytes input; double_data output
function double_data = bytes_uint8_to_double(bytes)

double_data    = zeros(1, 1, 'double');    % 明示的に型とサイズを宣言
unsigned_int   = typecast(uint8(bytes), 'uint32');
signed_int     = typecast(unsigned_int, 'int32');
double_data(1) = double(signed_int);       % サイズを明示

== matlab function roller485lib/Basic I2C Write (using MATLAB Function)/speed PID (using MATLAB Function)/MATLAB Function (I) ==
  data: double_data input; bytes output
function bytes = double_to_bytes_uint8(double_data)

bytes        = zeros(1, 4, 'uint8');             % 明示的に型とサイズを宣言
signed_int   = int32(double_data);
unsigned_int = typecast(signed_int, 'uint32');
bytes(1:4)   = typecast(unsigned_int, 'uint8');  % サイズを明示

== matlab function roller485lib/Basic I2C Write (using MATLAB Function)/speed PID (using MATLAB Function)/MATLAB Function (P) ==
  data: double_data input; bytes output
function bytes = double_to_bytes_uint8(double_data)

bytes        = zeros(1, 4, 'uint8');             % 明示的に型とサイズを宣言
signed_int   = int32(double_data);
unsigned_int = typecast(signed_int, 'uint32');
bytes(1:4)   = typecast(unsigned_int, 'uint8');  % サイズを明示

== matlab function roller485lib/Basic I2C Write (using MATLAB Function)/speed PID (within set time) (using MATLAB Function)/Enabled Subsystem/MATLAB Function (D) ==
  data: double_data input; bytes output
function bytes = double_to_bytes_uint8(double_data)

bytes        = zeros(1, 4, 'uint8');             % 明示的に型とサイズを宣言
signed_int   = int32(double_data);
unsigned_int = typecast(signed_int, 'uint32');
bytes(1:4)   = typecast(unsigned_int, 'uint8');  % サイズを明示

== matlab function roller485lib/Basic I2C Write (using MATLAB Function)/speed PID (within set time) (using MATLAB Function)/Enabled Subsystem/MATLAB Function (I) ==
  data: double_data input; bytes output
function bytes = double_to_bytes_uint8(double_data)

bytes        = zeros(1, 4, 'uint8');             % 明示的に型とサイズを宣言
signed_int   = int32(double_data);
unsigned_int = typecast(signed_int, 'uint32');
bytes(1:4)   = typecast(unsigned_int, 'uint8');  % サイズを明示

== matlab function roller485lib/Basic I2C Write (using MATLAB Function)/speed PID (within set time) (using MATLAB Function)/Enabled Subsystem/MATLAB Function (P) ==
  data: double_data input; bytes output
function bytes = double_to_bytes_uint8(double_data)

bytes        = zeros(1, 4, 'uint8');             % 明示的に型とサイズを宣言
signed_int   = int32(double_data);
unsigned_int = typecast(signed_int, 'uint32');
bytes(1:4)   = typecast(unsigned_int, 'uint8');  % サイズを明示

== matlab function roller485lib/I2C Write (using MATLAB Function)/angular velocity command [rpm] (using MATLAB Function)/Enabled Subsystem (PID setting)/MATLAB Function (P) ==
  data: double_data input; bytes output
function bytes = double_to_bytes_uint8(double_data)

bytes        = zeros(1, 4, 'uint8');             % 明示的に型とサイズを宣言
signed_int   = int32(double_data);
unsigned_int = typecast(signed_int, 'uint32');
bytes(1:4)   = typecast(unsigned_int, 'uint8');  % サイズを明示

== matlab function roller485lib/I2C Write (using MATLAB Function)/angular velocity command [rad//s] (using MATLAB Function)/Enabled Subsystem (PID setting)/MATLAB Function (D) ==
  data: double_data input; bytes output
function bytes = double_to_bytes_uint8(double_data)

bytes        = zeros(1, 4, 'uint8');             % 明示的に型とサイズを宣言
signed_int   = int32(double_data);
unsigned_int = typecast(signed_int, 'uint32');
bytes(1:4)   = typecast(unsigned_int, 'uint8');  % サイズを明示

== matlab function roller485lib/I2C Write (using MATLAB Function)/angular velocity command [rad//s] (using MATLAB Function)/Enabled Subsystem (PID setting)/MATLAB Function (I) ==
  data: double_data input; bytes output
function bytes = double_to_bytes_uint8(double_data)

bytes        = zeros(1, 4, 'uint8');             % 明示的に型とサイズを宣言
signed_int   = int32(double_data);
unsigned_int = typecast(signed_int, 'uint32');
bytes(1:4)   = typecast(unsigned_int, 'uint8');  % サイズを明示

== matlab function roller485lib/I2C Write (using MATLAB Function)/angular velocity command [rad//s] (using MATLAB Function)/Enabled Subsystem (PID setting)/MATLAB Function (P) ==
  data: double_data input; bytes output
function bytes = double_to_bytes_uint8(double_data)

bytes        = zeros(1, 4, 'uint8');             % 明示的に型とサイズを宣言
signed_int   = int32(double_data);
unsigned_int = typecast(signed_int, 'uint32');
bytes(1:4)   = typecast(unsigned_int, 'uint8');  % サイズを明示

== matlab function roller485lib/I2C Write (using MATLAB Function)/absolute angle command [deg] (using MATLAB Function)/Enabled Subsystem (PID setting)/MATLAB Function (D) ==
  data: double_data input; bytes output
function bytes = double_to_bytes_uint8(double_data)

bytes        = zeros(1, 4, 'uint8');             % 明示的に型とサイズを宣言
signed_int   = int32(double_data);
unsigned_int = typecast(signed_int, 'uint32');
bytes(1:4)   = typecast(unsigned_int, 'uint8');  % サイズを明示

== matlab function roller485lib/Basic I2C Write (using MATLAB Function)/basic absolute angle command [deg] (using MATLAB Function)/MATLAB Function ==
  data: double_data input; bytes output
function bytes = double_to_bytes_uint8(double_data)

bytes        = zeros(1, 4, 'uint8');             % 明示的に型とサイズを宣言
signed_int   = int32(double_data);
unsigned_int = typecast(signed_int, 'uint32');
bytes(1:4)   = typecast(unsigned_int, 'uint8');  % サイズを明示

== matlab function roller485lib/I2C Write (using MATLAB Function)/absolute angle command [deg] (using MATLAB Function)/Enabled Subsystem (PID setting)/MATLAB Function (I) ==
  data: double_data input; bytes output
function bytes = double_to_bytes_uint8(double_data)

bytes        = zeros(1, 4, 'uint8');             % 明示的に型とサイズを宣言
signed_int   = int32(double_data);
unsigned_int = typecast(signed_int, 'uint32');
bytes(1:4)   = typecast(unsigned_int, 'uint8');  % サイズを明示
